simulink model "test_entkopplung"  (R2020a)
settings: Solver=VariableStepAuto  StartTime=0.0  StopTime=3800  RelTol=1e-3
libraries: simulink x7, library_schuettgut x1
settings Model: Creator=Jonathan  LastModifiedBy=Jonathan

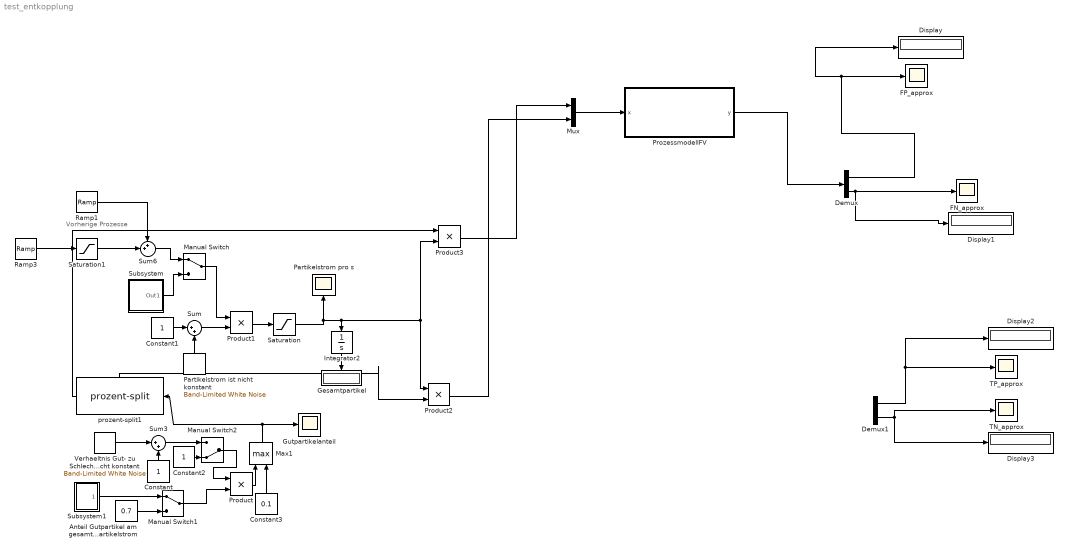
== system test_entkopplung ==
  note: Vorherige Prozesse
  Anteil Gutpartikel am gesamten Partikelstrom : Constant  Value=0.7
  Constant : Constant
  Constant1 : Constant
  Constant2 : Constant
  Constant3 : Constant  Value=0.1
  Demux : Demux  Outputs=2
  Demux1 : Demux  Outputs=2
  Display{,1..3} (4 alike) : Display
  FN_approx : Scope
  FP_approx : Scope
  Gesamtpartikel : Display
  Gutpartikelanteil : Scope
  Integrator2 : Integrator
  Manual Switch : ManualSwitch
  Manual Switch1 : ManualSwitch
  Manual Switch2 : ManualSwitch  CurrentSetting=0
  Max1 : MinMax  Function=max  Inputs=2
  Mux : Mux  Inputs=2
  Partikelstrom ist nicht konstant : simulink/Sources/Band-Limited White Noise  Cov=[0.00001]  Ts=0.1  seed=[23341]
  Partikelstrom pro s : Scope
  Product{,1..3} (4 alike) : Product
  ProzessmodellFV : Subsystem  AncestorBlock=library_schuettgut/ProzessmodellFV
  Ramp1 : simulink/Sources/Ramp  slope=-1 * 3/200  start=3600-300  InitialOutput=0
  Ramp3 : simulink/Sources/Ramp  slope=0.01  start=0  InitialOutput=0
  Saturation : Saturate  UpperLimit=20  LowerLimit=0
  Saturation1 : Saturate  UpperLimit=3  LowerLimit=0
  Subsystem : Subsystem
  Subsystem1 : Subsystem
  Sum : Sum  Inputs=|++
  Sum3 : Sum  Inputs=|++
  Sum6 : Sum  Inputs=++|
  TN_approx : Scope
  TP_approx : Scope
  Verhaeltnis Gut- zu Schlechtpartikel ist nicht konstant : simulink/Sources/Band-Limited White Noise  Cov=[0.00001]  Ts=0.1  seed=[13341]
  prozent-split1 : library_schuettgut/prozent-split  SystemSampleTime=-1  SSRTWFcnClass=[]  Latency=0  AutoFrameSizeCalculation=off
      settings: PortSchema="{\"entries\":[{\"content\":{\"sides\":[{\"content\":{\"connectorIds\":[\"In1\"]},\"type\":\"ConnectorPlacement.EquallySpacedRectSide\",\"uuid\":\"ab8511c8-9f1d-48ad-bf24-85fd477f0bdd\"},{\"content\":{\"connectorIds\":[\"Out1\"],\"side\":\"RIGHT\"},\"type\":\"ConnectorPlacement.EquallySpacedRectSide\",\"uuid\":\"9ac1a19a-8176-444e-9f4d-7beffa0184e3\"},{\"content\":{\"connectorIds\":[\"Out2\"],\"side\":\"TOP\"},\"type\":\"ConnectorPlacement.EquallySpacedRectSide\",\"uuid\":\"376c2400-f821-4649-ab16-706a2da6117b\"}]},\"type\":\"ConnectorPlacement.EquallySpacedConnector\",\"uuid\":\"f6e72b2d-0467-4732-a018-d51f3a5db703\"}],\"packageUris\":[\"http://schema.mathworks.com/mf0/Connector/19700101\"],\"version\":\"1.0\"}"
  wires:
  ProzessmodellFV/1(y) -> Demux/1
  Demux/1 -> Display/1, FP_approx/1
  Demux/2 -> Display1/1, FN_approx/1
  Mux/1 -> ProzessmodellFV/1(x)
  Demux1/1 -> Display2/1, TP_approx/1
  ? -> Demux1/1
  Demux1/2 -> TN_approx/1, Display3/1
  Ramp3/1 -> Saturation1/1
  Sum3/1 -> Manual Switch2/1
  Subsystem/1(Out1) -> Manual Switch/2
  Manual Switch/1 -> Product1/1
  Partikelstrom ist nicht konstant/1 -> Sum/2
  Product/1 -> Max1/1
  Ramp1/1 -> Sum6/1
  Constant3/1 -> Max1/2
  Max1/1 -> prozent-split1/1, Gutpartikelanteil/1
  Constant2/1 -> Manual Switch2/2
  Anteil Gutpartikel am gesamten Partikelstrom/1 -> Manual Switch1/2
  Integrator2/1 -> Gesamtpartikel/1
  Sum/1 -> Product1/2
  Manual Switch2/1 -> Product/1
  Constant1/1 -> Sum/1
  Sum6/1 -> Manual Switch/1
  prozent-split1/2 -> Product2/2
  Product2/1 -> Mux/2
  Verhaeltnis Gut- zu Schlechtpartikel ist nicht konstant/1 -> Sum3/1
  Saturation1/1 -> Sum6/2
  Subsystem1/1(Out1) -> Manual Switch1/1
  Manual Switch1/1 -> Product/2
  Constant/1 -> Sum3/2
  Saturation/1 -> Product2/1, Product3/2, Integrator2/1, Partikelstrom pro s/1
  Product1/1 -> Saturation/1
  prozent-split1/1 -> Product3/1
  Product3/1 -> Mux/1

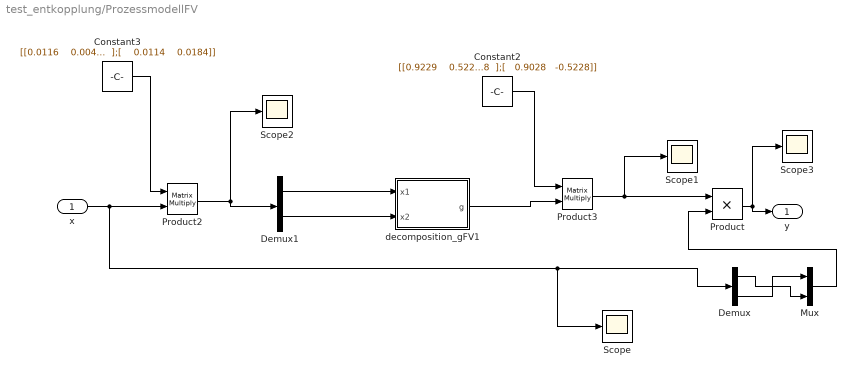
== system test_entkopplung/ProzessmodellFV ==
  x : Inport
  Constant2 : Constant  Value=|
      | [[0.9229    0.5228
      |  ];[   0.9028   -0.5228]]
  Constant3 : Constant  Value=|  VectorParams1D=off
      | [[0.0116    0.0046
      |  ];[    0.0114    0.0184]]
  Demux : Demux  Outputs=2
  Demux1 : Demux  Outputs=2
  Mux : Mux  Inputs=2
  Product : Product
  Product2 : Product  Multiplication=Matrix(*)
  Product3 : Product  Multiplication=Matrix(*)
  Scope{,1..3} (4 alike) : Scope
  decomposition_gFV1 : MATLAB Function  AncestorBlock=library_schuettgut/decomposition_gFV  TreatAsAtomicUnit=on
  y : Outport
  wires:
  x/1 -> Demux/1, Scope/1, Product2/2
  decomposition_gFV1/1(g) -> Product3/2
  Demux1/1 -> decomposition_gFV1/1(x1)
  Demux1/2 -> decomposition_gFV1/2(x2)
  Constant2/1 -> Product3/1
  Product3/1 -> Scope1/1, Product/1
  Product2/1 -> Scope2/1, Demux1/1
  Constant3/1 -> Product2/1
  Product/1 -> y/1, Scope3/1
  Demux/2 -> Mux/1
  Demux/1 -> Mux/2
  Mux/1 -> Product/2

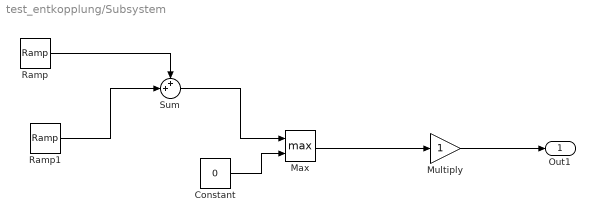
== system test_entkopplung/Subsystem ==
  Constant : Constant  Value=0
  Max : MinMax  Function=max  Inputs=2
  Multiply : Gain
  Ramp : simulink/Sources/Ramp  slope=10  start=0  InitialOutput=0
  Ramp1 : simulink/Sources/Ramp  slope=-20  start=100  InitialOutput=0
  Sum : Sum  Inputs=++|
  Out1 : Outport
  wires:
  Max/1 -> Multiply/1
  Constant/1 -> Max/2
  Sum/1 -> Max/1
  Ramp1/1 -> Sum/2
  Ramp/1 -> Sum/1
  Multiply/1 -> Out1/1

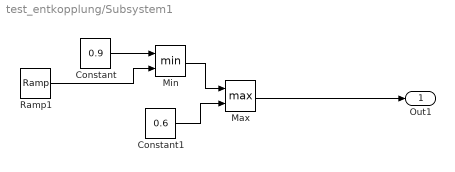
== system test_entkopplung/Subsystem1 ==
  Constant : Constant  Value=0.9
  Constant1 : Constant  Value=0.6
  Max : MinMax  Function=max  Inputs=2
  Min : MinMax  Inputs=2
  Ramp1 : simulink/Sources/Ramp  slope=-0.03  start=500  InitialOutput=0.8
  Out1 : Outport
  wires:
  Max/1 -> Out1/1
  Constant/1 -> Min/1
  Constant1/1 -> Max/2
  Min/1 -> Max/1
  Ramp1/1 -> Min/2

== matlab function test_entkopplung/ProzessmodellFV/decomposition_gFV1 ==
  data: x1 input; g output; x2 input
function g = decomposition_gFV(x1,x2)
%#codegen

%    This function was generated by the Symbolic Math Toolbox version 8.5.
%    26-Jan-2021 22:17:03

g = [conj(x1).*(-1.377937986499028e-2)+1.601570395857327e-1;conj(x2).*1.81125395555236e-2+8.513571412265965e-2];
